simulink model "FM_system"  (R2019b)
settings: Solver=VariableStepAuto  StartTime=0.0  StopTime=2  RelTol=1e-3
libraries: dsparch4 x1, commsynccomp2 x1
settings Model: Creator=SEFA  LastModifiedBy=SEFA

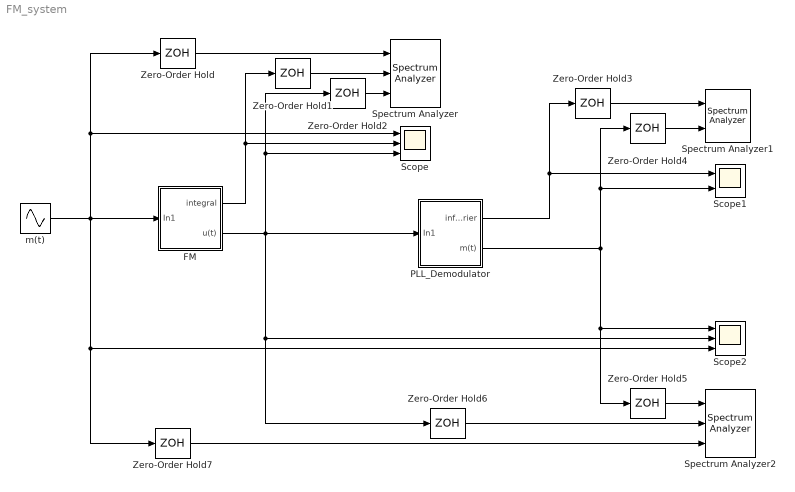
== system FM_system ==
  FM : Subsystem
  PLL_Demodulator : Subsystem
  Scope : Scope  NumInputPorts=3
  Scope1 : Scope  NumInputPorts=2
  Scope2 : Scope  NumInputPorts=3
  Spectrum Analyzer : SpectrumAnalyzer  NumInputPorts=3
  Spectrum Analyzer1 : SpectrumAnalyzer  NumInputPorts=2
  Spectrum Analyzer2 : SpectrumAnalyzer  NumInputPorts=3
  Zero-Order Hold{,1..2,5..7} (6 alike) : ZeroOrderHold  SampleTime=5e-4
  Zero-Order Hold3 : ZeroOrderHold  SampleTime=5/10000
  Zero-Order Hold4 : ZeroOrderHold  SampleTime=5/10000
  m(t) : Sin  Amplitude=-1  Frequency=2*pi*50  SampleTime=1e-5
  wires:
  m(t)/1 -> Zero-Order Hold7/1, Scope2/3, Scope/1, Zero-Order Hold/1, FM/1(In1)
  FM/2(u(t)) -> Scope2/2, Zero-Order Hold6/1, Zero-Order Hold2/1, Scope/3, PLL_Demodulator/1(In1)
  FM/1(integral) -> Zero-Order Hold1/1, Scope/2
  Zero-Order Hold/1 -> Spectrum Analyzer/1
  Zero-Order Hold1/1 -> Spectrum Analyzer/2
  Zero-Order Hold2/1 -> Spectrum Analyzer/3
  Zero-Order Hold3/1 -> Spectrum Analyzer1/1
  Zero-Order Hold4/1 -> Spectrum Analyzer1/2
  PLL_Demodulator/2(m(t)) -> Zero-Order Hold5/1, Scope2/1, Scope1/2, Zero-Order Hold4/1
  PLL_Demodulator/1(info_carrier) -> Zero-Order Hold3/1, Scope1/1
  Zero-Order Hold5/1 -> Spectrum Analyzer2/1
  Zero-Order Hold7/1 -> Spectrum Analyzer2/3
  Zero-Order Hold6/1 -> Spectrum Analyzer2/2

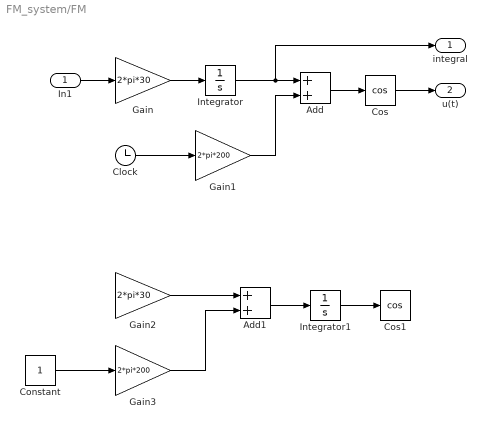
== system FM_system/FM ==
  In1 : Inport
  Add : Sum
  Add1 : Sum
  Clock : Clock
  Constant : Constant
  Cos : Trigonometry  Operator=cos
  Cos1 : Trigonometry  Operator=cos
  Gain : Gain  Gain=2*pi*30
  Gain1 : Gain  Gain=2*pi*200
  Gain2 : Gain  Gain=2*pi*30
  Gain3 : Gain  Gain=2*pi*200
  Integrator : Integrator  InitialCondition=3/5
  Integrator1 : Integrator  InitialCondition=3/5
  integral : Outport
  u(t) : Outport  Port=2
  wires:
  Clock/1 -> Gain1/1
  Gain1/1 -> Add/2
  In1/1 -> Gain/1
  Integrator/1 -> integral/1, Add/1
  Gain/1 -> Integrator/1
  Add/1 -> Cos/1
  Gain2/1 -> Add1/1
  Constant/1 -> Gain3/1
  Gain3/1 -> Add1/2
  Add1/1 -> Integrator1/1
  Integrator1/1 -> Cos1/1
  Cos/1 -> u(t)/1

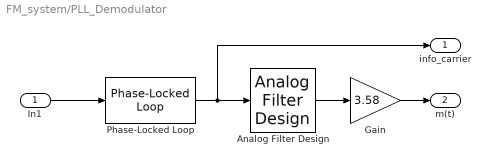
== system FM_system/PLL_Demodulator ==
  In1 : Inport
  Analog Filter Design : dsparch4/Analog Filter Design  method=Butterworth  filttype=Lowpass  N=8  Wlo=2*pi*60  Whi=80  Rp=2  Rs=40
  Gain : Gain  Gain=3.58
  Phase-Locked Loop : commsynccomp2/Phase-Locked Loop  Fn="[3.0002  0  40002]"  Fd="[1   67.46   2270.9   40002]"  Kvco=1  Fc=200  Ph=pi/2  Ac=1
      settings: SourceProductName=Communications Toolbox  SourceProductBaseCode=CM
  info_carrier : Outport
  m(t) : Outport  Port=2
  wires:
  Gain/1 -> m(t)/1
  Analog Filter Design/1 -> Gain/1
  In1/1 -> Phase-Locked Loop/1
  Phase-Locked Loop/2 -> info_carrier/1, Analog Filter Design/1
